simulink subsystem "predictor_2021b"  (R2021b)
settings: Solver=VariableStepAuto  StartTime=0.0  StopTime=10.0  RelTol=1e-3
settings Model: Creator=marin  LastModifiedBy=local_adm
settings DebuggingCC: UnconnectedInputMsg=none  UnconnectedOutputMsg=none  UnconnectedLineMsg=none
settings ModelReferenceCC: EnableRefExpFcnMdlSchedulingChecks=off
settings RTWCC: DLArmComputeVersion=20.02.1

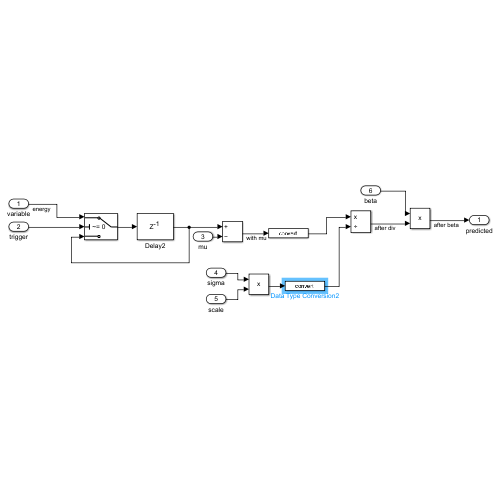
[thumbnail: Simulink's stored preview of the top-level diagram]
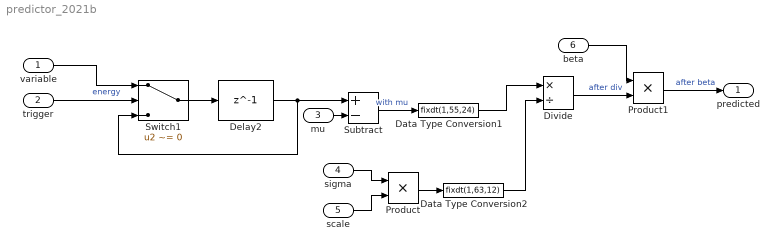
== system predictor_2021b ==
  variable : Inport
  trigger : Inport  Port=2
  mu : Inport  Port=3
  sigma : Inport  Port=4
  scale : Inport  Port=5
  beta : Inport  Port=6
  Data Type Conversion1 : DataTypeConversion  OutMax=2  OutDataTypeStr=fixdt(1,55,24)
  Data Type Conversion2 : DataTypeConversion  OutMax=2  OutDataTypeStr=fixdt(1,63,12)
  Delay2 : Delay  DelayLength=1  InitialCondition=0  UseCircularBuffer=on
  Divide : Product  Inputs=*/  OutDataTypeStr=fixdt(1,42,12)  RndMeth=Zero  SaturateOnIntegerOverflow=on
  Product : Product
  Product1 : Product  OutDataTypeStr=fixdt(1,32,12)
  Subtract : Sum  Inputs=+-
  Switch1 : Switch  Criteria=u2 ~= 0
  predicted : Outport
  wires:
  variable/1 -> Switch1/1  "energy"
  Divide/1 -> Product1/2  "after div"
  trigger/1 -> Switch1/2
  Delay2/1 -> Switch1/3, Subtract/1
  Switch1/1 -> Delay2/1
  Product1/1 -> predicted/1  "after beta"
  mu/1 -> Subtract/2
  sigma/1 -> Product/1
  scale/1 -> Product/2
  beta/1 -> Product1/1
  Subtract/1 -> Data Type Conversion1/1  "with mu"
  Data Type Conversion1/1 -> Divide/1
  Product/1 -> Data Type Conversion2/1
  Data Type Conversion2/1 -> Divide/2
